simulink model "FatigueTesting"  (R2012b)
settings: Solver=ode1  StartTime=0.0  StopTime=tend  FixedStep=0.001  RelTol=1e-3
undefined symbols (not defined in the file): dtr, dtw, HIL, LCconv, Nr, Nw, ptw, sat, tfat, thresh
libraries: quarc_library x3, ScienceStimHasomed_Lib x1, simulink x1
settings Model: SimulationMode=external  ExtModeTrigDuration=5000000  Creator=LabUser  LastModifiedBy=LabUser
settings SolverCC: PositivePriorityOrder=on
settings DataIOCC: LimitDataPoints=off
settings DebuggingCC: SolverPrmCheckMsg=none
settings RTWCC: SystemTargetFile=quarc_win64.tlc  TemplateMakefile=quarc_default_tmf  Description=QUARC Win64 Target  ProcessScript=quarc_win64_make_rtw_hook
settings RTWCC: CustomLibrary=|
  | sciencemode.obj
  | serial_windows.obj
settings STFCustomTargetCC: TargetPreCompLibLocation=C:\PROGRA~3\QUARC\lib\2012b\win64\release  CodeReplacementLibrary=ANSI_C  GeneratePreprocessorConditionals=Disable all  CombineOutputUpdateFcns=on  GRTInterface=off  SystemTargetFile=quarc_win64.tlc
settings GRTTargetCC: TargetPreCompLibLocation=C:\PROGRA~3\QUARC\lib\2012b\win64\release  ParMdlRefBuildCompliant=off  CompOptLevelCompliant=off  ConcurrentExecutionCompliant=off  MatFileLogging=off  ExtMode=on  ExtModeMexFile=quarc_comm

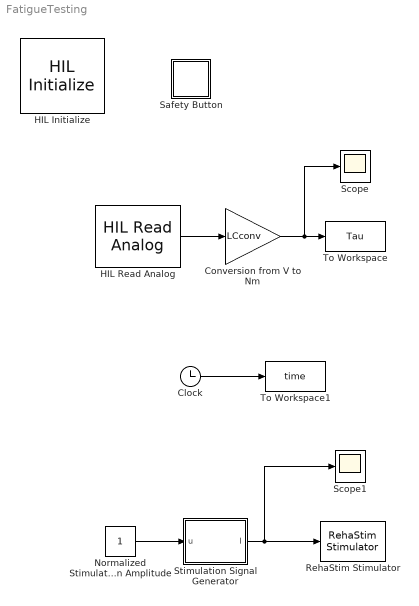
== system FatigueTesting ==
  Clock : Clock
  Conversion from V to Nm : Gain  Gain=LCconv
  HIL Initialize : quarc_library/Data Acquisition/Generic/Configuration/HIL Initialize  Priority=-99  object_name=HIL-1  board_type=qpid_e  board_number=0  board_options=enc0_dir=0;enc0_filter=1;enc0_a=1;enc0_b=1;enc0_z=0;enc0_reload=0;enc1_dir=0;enc1_filter=1;enc1_a=1;enc1_b=1;enc1_z=0;enc1_reload=0;enc2_dir=0;enc2_filter=1;enc2_a=1;enc2_b=1;enc2_z=0;enc2_reload=0;enc3_dir=0;enc3_filter=1;enc3_a=1;enc3_b=1;enc3_z=0;enc3_reload=0;enc4_dir=0;enc4_filter=1;enc4_a=1;enc4_b=1;enc4_z=0;enc4_reload=0;enc5_dir=0;enc5_filter=1;enc5_a=1;enc5_b=1;enc5_z=0;enc5_reload=0;enc6_dir=0;enc6_filter=1;enc6_a=1;enc6_b=1;enc6_z=0;enc6_reload=0;enc7_dir=0;enc7_filter=1;enc7_a=1;enc7_b=1;enc7_z=0;enc7_reload=0;ext_int_polarity=0;fuse_polarity=0;convert_polarity=0;watchdog_polarity=0;ext_int_watchdog=0;fuse_watchdog=0;trig1_watchdog=0;watchdog_to_trig1=0;watchdog_to_trig2=0;counter_to_trig0=0;trigger_adcs=0;latch_on_adc=0;pwm_immediate=0  exclusive=off  active=off  hardware_clocks=[0:16]  clock_modes=[]  initial_clock_frequencies=[]  set_clock_params_at_start=off  set_clock_params_at_switch_in=off  set_clock_frequencies_at_start=off  set_clock_frequencies_at_switch_in=off  analog_input_channels=[0:7]  analog_input_maximums=10  analog_input_minimums=-10  set_analog_input_params_at_start=off  set_analog_input_params_at_switch_in=off  analog_output_channels=[0:7]  analog_output_maximums=10  analog_output_minimums=-10  initial_analog_outputs=[0]  final_analog_outputs=[0]  watchdog_analog_outputs=0  set_analog_output_params_at_start=off  set_analog_output_params_at_switch_in=off  set_analog_outputs_at_start=on  set_analog_outputs_at_switch_in=off  set_analog_outputs_at_terminate=on  set_analog_outputs_at_switch_out=off  set_analog_outputs_on_watchdog=off  digital_input_channels=[]  digital_output_channels=[]  digital_output_configuration=[]  initial_digital_outputs=[1]  final_digital_outputs=[1]  watchdog_digital_outputs=[2]  set_digital_output_params_at_start=off  set_digital_output_params_at_switch_in=off  set_digital_outputs_at_start=on  set_digital_outputs_at_switch_in=off  set_digital_outputs_at_terminate=on  set_digital_outputs_at_switch_out=off  set_digital_outputs_on_watchdog=off  encoder_channels=[0:7]  quadrature=[4]  encoder_filter_frequency=40e6/1  initial_encoder_counts=[0]  set_encoder_params_at_start=on  set_encoder_params_at_switch_in=off  set_encoder_counts_at_start=off  set_encoder_counts_at_switch_in=off  pwm_channels=[0:7]  pwm_modes=0  pwm_frequency=40e6/4096  pwm_configuration=[0]  pwm_alignment=[0]  pwm_polarity=[1]  pwm_leading_deadband=[0]  pwm_trailing_deadband=[0]  initial_pwm_outputs=[0]  final_pwm_outputs=[0]  watchdog_pwm_outputs=[0]  set_pwm_params_at_start=on  set_pwm_params_at_switch_in=off  set_pwm_outputs_at_start=on  set_pwm_outputs_at_switch_in=off  set_pwm_outputs_at_terminate=on  set_pwm_outputs_at_switch_out=off  set_pwm_outputs_on_watchdog=off  other_output_channels=[]  initial_other_outputs=[]  final_other_outputs=[]  watchdog_other_outputs=[]  set_other_outputs_at_start=off  set_other_outputs_at_switch_in=off  set_other_outputs_at_terminate=off  set_other_outputs_at_switch_out=off  set_other_outputs_on_watchdog=off
  HIL Read Analog : quarc_library/Data Acquisition/Generic/Immediate I//O/HIL Read Analog  object_name=HIL-1  channels=0  sample_time=qc_get_step_size  active=on  vector_output=off
  Normalized Stimulation Amplitude : Constant
  RehaStim Stimulator : ScienceStimHasomed_Lib/RehaStim Stimulator  sFreq=1000  Freq=stimfreq  PWidth=PW
  Safety Button : Subsystem
  Scope : Scope
      settings: YMin=0  YMax=95  MaxDataPoints=500000
  Scope1 : Scope
      settings: YMin=0  YMax=65000  MaxDataPoints=500000
  Stimulation Signal Generator : Subsystem  mask{Nw=Nw, tfat=tfat, Nr=Nr, dtw=dtw, dtr=dtr, ptw=ptw}
      mask prompts: Nw "Number of warmup pulses:"; tfat "Duration of fatiguing stimulation [s]:"; Nr "Number of recovery pulses:"; dtw "Time between warmup pulses [s]:"; dtr "Time between recovery pulses [s]:"; ptw "Duration of warmup and recovery pulses [s]:"
  To Workspace : ToWorkspace  VariableName=Tau  SampleTime=-1
  To Workspace1 : ToWorkspace  VariableName=time  SampleTime=-1
  wires:
  HIL Read Analog/1 -> Conversion from V to Nm/1
  Conversion from V to Nm/1 -> Scope/1, To Workspace/1
  Clock/1 -> To Workspace1/1
  Normalized Stimulation Amplitude/1 -> Stimulation Signal Generator/1(u)
  Stimulation Signal Generator/1(I) -> RehaStim Stimulator/1, Scope1/1

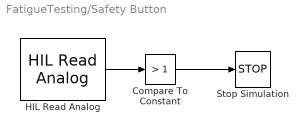
== system FatigueTesting/Safety Button ==
  Compare To Constant : simulink/Logic and Bit Operations/Compare To Constant  relop=>  const=1  OutDataTypeStr=boolean
  HIL Read Analog : quarc_library/Data Acquisition/Generic/Immediate I//O/HIL Read Analog  object_name=HIL-1  channels=[7]  sample_time=qc_get_step_size  active=on  vector_output=off
  Stop Simulation : Stop
  wires:
  HIL Read Analog/1 -> Compare To Constant/1
  Compare To Constant/1 -> Stop Simulation/1

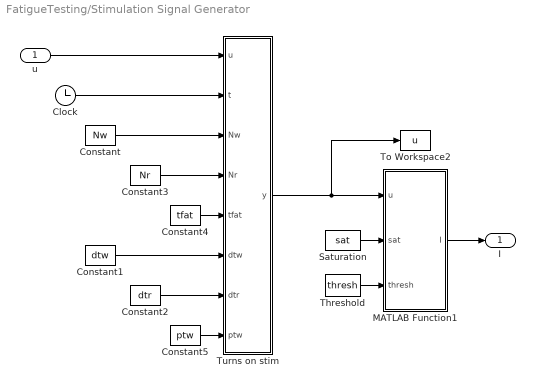
== system FatigueTesting/Stimulation Signal Generator ==
  u : Inport
  Clock : Clock
  Constant : Constant  Value=Nw
  Constant1 : Constant  Value=dtw
  Constant2 : Constant  Value=dtr
  Constant3 : Constant  Value=Nr
  Constant4 : Constant  Value=tfat
  Constant5 : Constant  Value=ptw
  MATLAB Function1 : MATLAB Function  TreatAsAtomicUnit=on
  Saturation : Constant  Value=sat
  Threshold : Constant  Value=thresh
  To Workspace2 : ToWorkspace  VariableName=u  SampleTime=-1
  Turns on stim : MATLAB Function  TreatAsAtomicUnit=on
  I : Outport
  wires:
  u/1 -> Turns on stim/1(u)
  Clock/1 -> Turns on stim/2(t)
  MATLAB Function1/1(I) -> I/1
  Saturation/1 -> MATLAB Function1/2(sat)
  Threshold/1 -> MATLAB Function1/3(thresh)
  Constant/1 -> Turns on stim/3(Nw)
  Constant4/1 -> Turns on stim/5(tfat)
  Constant3/1 -> Turns on stim/4(Nr)
  Turns on stim/1(y) -> To Workspace2/1, MATLAB Function1/1(u)
  Constant1/1 -> Turns on stim/6(dtw)
  Constant2/1 -> Turns on stim/7(dtr)
  Constant5/1 -> Turns on stim/8(ptw)

== matlab function FatigueTesting/Stimulation Signal Generator/MATLAB Function1 ==
  data: u input; I output; sat input; thresh input
function I = fcn(u,sat,thresh)

if u <= 0
    I = 0;
elseif u >= 1
    I = sat;
else
    I = thresh + u*(sat-thresh);
end

== matlab function FatigueTesting/Stimulation Signal Generator/Turns on stim ==
  data: u input; y output; t input; Nw input; Nr input; tfat input; dtw input; dtr input; ptw input
function y = fcn(u,t,Nw,Nr,tfat,dtw,dtr,ptw)


%% Stimulation Pulse Logic

% Total time for warmup
tw = Nw*(dtw+ptw);
% Warmup start time
twstart = 5;

% Fatigue start time
tfstart = twstart+tw+dtw;

% Total time for recovery pulses
tr = Nr*(dtr+ptw);
% Recovery start time
trstart = tfstart+tfat;

NNw = 1:10;
NNr = 1:10;

if (t >= twstart) && (t <= twstart+tw)
    % This is the time when the warmup stimulation is applied.
    trel = t-twstart;
    
    if any((trel >= (NNw-1)*ptw+NNw*dtw) + (trel <= NNw*(dtw+ptw)) == 2)
        y = u;
    else
        y = 0;
    end
    
elseif (t >= tfstart) && (t <= tfstart+tfat)
    % This is the time period when the muslces are beign constantly
    % stimulated.
    y = u;
    
elseif (t > trstart) && (t <= trstart+tr)
    % this is the recovery period.
    trel = t-trstart;
    
    if any((trel >= (NNr-1)*ptw+NNr*dtr) + (trel <= NNr*(dtr+ptw)) == 2)
        y = u;
    else
        y = 0;
    end
    
else
    % Otherwise do not output a stimulation.
    y = 0;
end
